simulink model "hpa_module"  (R2019a)
settings: Solver=FixedStepDiscrete  StartTime=0.0  StopTime=inf  RelTol=1e-3
InitFcn:
  | f = 300e6;
libraries: hdlsllib x5, simulink x1
settings Model: DataTypeOverride=Off  Creator=David Northcote  LastModifiedBy=David Northcote
settings DataIOCC: SaveOutput=off  SaveTime=off
settings OptimizationCC: BlockReduction=off  ConditionallyExecuteInputs=off  DefaultParameterBehavior=Inlined
settings DebuggingCC: AlgebraicLoopMsg=error  SingleTaskRateTransMsg=error
settings HardwareCC: ProdBitPerPointer=32  ProdBitPerSizeT=32  ProdBitPerPtrDiffT=32  ProdLargestAtomicFloat=None  ProdIntDivRoundTo=Undefined  ProdEndianess=Unspecified  ProdWordSize=32  ProdHWDeviceType=ASIC/FPGA->ASIC/FPGA  TargetBitPerPointer=64  TargetBitPerSizeT=64  TargetBitPerPtrDiffT=64  TargetLongLongMode=on  TargetIntDivRoundTo=Zero  TargetEndianess=LittleEndian  TargetWordSize=64  TargetHWDeviceType=Custom Processor->MATLAB Host Computer  ProdEqTarget=off

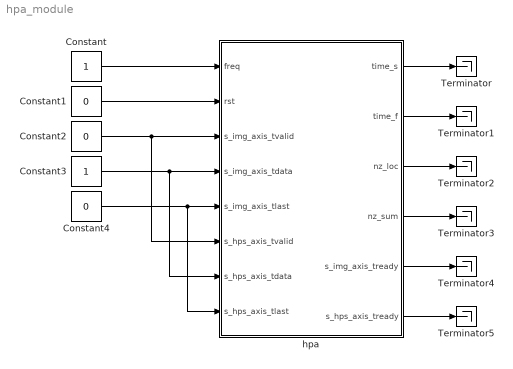
== system hpa_module ==
  Constant : Constant  OutDataTypeStr=uint32  SampleTime=1/f
  Constant1 : Constant  Value=0  OutDataTypeStr=boolean  SampleTime=1/f
  Constant2 : Constant  Value=0  OutDataTypeStr=boolean  SampleTime=1/f
  Constant3 : Constant  OutDataTypeStr=uint32  SampleTime=1/f
  Constant4 : Constant  Value=0  OutDataTypeStr=boolean  SampleTime=1/f
  Terminator{,1..5} (6 alike) : Terminator
  hpa : Subsystem  TreatAsAtomicUnit=on
  wires:
  Constant/1 -> hpa/1(freq)
  Constant1/1 -> hpa/2(rst)
  Constant2/1 -> hpa/6(s_hps_axis_tvalid), hpa/3(s_img_axis_tvalid)
  Constant3/1 -> hpa/7(s_hps_axis_tdata), hpa/4(s_img_axis_tdata)
  Constant4/1 -> hpa/8(s_hps_axis_tlast), hpa/5(s_img_axis_tlast)
  hpa/1(time_s) -> Terminator/1
  hpa/2(time_f) -> Terminator1/1
  hpa/3(nz_loc) -> Terminator2/1
  hpa/4(nz_sum) -> Terminator3/1
  hpa/6(s_hps_axis_tready) -> Terminator5/1
  hpa/5(s_img_axis_tready) -> Terminator4/1

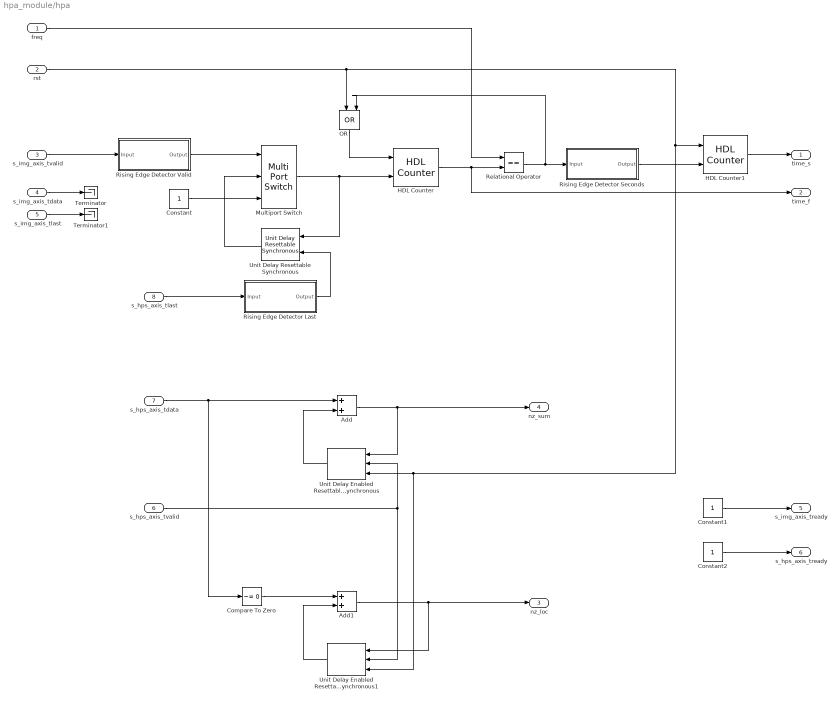
== system hpa_module/hpa ==
  freq : Inport
  rst : Inport  Port=2
  s_img_axis_tvalid : Inport  Port=3
  s_img_axis_tdata : Inport  Port=4
  s_img_axis_tlast : Inport  Port=5
  s_hps_axis_tvalid : Inport  Port=6
  s_hps_axis_tdata : Inport  Port=7
  s_hps_axis_tlast : Inport  Port=8
  Add : Sum  OutDataTypeStr=uint32
  Add1 : Sum  OutDataTypeStr=uint32
  Compare To Zero : simulink/Logic and Bit Operations/Compare To Zero  relop=~=  OutDataTypeStr=boolean
  Constant : Constant  OutDataTypeStr=boolean  SampleTime=-1
  Constant1 : Constant  OutDataTypeStr=boolean  SampleTime=1/f
  Constant2 : Constant  OutDataTypeStr=boolean  SampleTime=1/f
  HDL Counter : hdlsllib/Sources/HDL Counter  CountType=Free running  CountInit=0  CountStep=1  CountMax=25  CountFromType=Initial value  CountFrom=0  CountResetPort=on  CountLoadPort=off  CountEnbPort=on  CountDirPort=off  CountDataType=Unsigned  CountWordLen=32  CountFracLen=0  CountSampTime=1
      settings: SourceProductName=Simulink
  HDL Counter1 : hdlsllib/Sources/HDL Counter  CountType=Free running  CountInit=0  CountStep=1  CountMax=25  CountFromType=Initial value  CountFrom=0  CountResetPort=on  CountLoadPort=off  CountEnbPort=on  CountDirPort=off  CountDataType=Unsigned  CountWordLen=32  CountFracLen=0  CountSampTime=1
      settings: SourceProductName=Simulink
  Multiport Switch : MultiPortSwitch  DataPortOrder=Zero-based contiguous  Inputs=2  zeroidx=on
  OR : Logic  Operator=OR  IconShape=distinctive  AllPortsSameDT=off  OutDataTypeStr=boolean
  Relational Operator : RelationalOperator  Operator===  OutDataTypeStr=boolean  RndMeth=Simplest
  Rising Edge Detector Last : Subsystem
  Rising Edge Detector Seconds : Subsystem
  Rising Edge Detector Valid : Subsystem
  Terminator : Terminator
  Terminator1 : Terminator
  Unit Delay Enabled Resettable Synchronous : hdlsllib/Discrete/Unit Delay Enabled Resettable Synchronous  InitialCondition=0.0  SampleTime=-1
      settings: SourceProductName=Simulink  SourceProductBaseCode=SL
  Unit Delay Enabled Resettable Synchronous1 : hdlsllib/Discrete/Unit Delay Enabled Resettable Synchronous  InitialCondition=0.0  SampleTime=-1
      settings: SourceProductName=Simulink  SourceProductBaseCode=SL
  Unit Delay Resettable Synchronous : hdlsllib/Discrete/Unit Delay Resettable Synchronous  InitialCondition=0.0  SampleTime=-1
      settings: SourceProductName=Simulink  SourceProductBaseCode=SL
  time_s : Outport
  time_f : Outport  Port=2
  nz_loc : Outport  Port=3
  nz_sum : Outport  Port=4
  s_img_axis_tready : Outport  Port=5
  s_hps_axis_tready : Outport  Port=6
  wires:
  Multiport Switch/1 -> HDL Counter/2, Unit Delay Resettable Synchronous/1
  s_hps_axis_tlast/1 -> Rising Edge Detector Last/1(Input)
  Unit Delay Resettable Synchronous/1 -> Multiport Switch/2
  Constant/1 -> Multiport Switch/3
  s_img_axis_tvalid/1 -> Rising Edge Detector Valid/1(Input)
  Rising Edge Detector Valid/1(Output) -> Multiport Switch/1
  Relational Operator/1 -> OR/2, Rising Edge Detector Seconds/1(Input)
  HDL Counter/1 -> time_f/1, Relational Operator/2
  freq/1 -> Relational Operator/1
  HDL Counter1/1 -> time_s/1
  s_img_axis_tdata/1 -> Terminator/1
  s_img_axis_tlast/1 -> Terminator1/1
  Rising Edge Detector Seconds/1(Output) -> HDL Counter1/2
  OR/1 -> HDL Counter/1
  s_hps_axis_tdata/1 -> Compare To Zero/1, Add/1
  Add/1 -> nz_sum/1, Unit Delay Enabled Resettable Synchronous/1
  Unit Delay Enabled Resettable Synchronous/1 -> Add/2
  s_hps_axis_tvalid/1 -> Unit Delay Enabled Resettable Synchronous/2, Unit Delay Enabled Resettable Synchronous1/2
  Unit Delay Enabled Resettable Synchronous1/1 -> Add1/2
  Add1/1 -> nz_loc/1, Unit Delay Enabled Resettable Synchronous1/1
  Compare To Zero/1 -> Add1/1
  rst/1 -> OR/1, Unit Delay Enabled Resettable Synchronous1/3, Unit Delay Enabled Resettable Synchronous/3, HDL Counter1/1
  Rising Edge Detector Last/1(Output) -> Unit Delay Resettable Synchronous/2
  Constant1/1 -> s_img_axis_tready/1
  Constant2/1 -> s_hps_axis_tready/1

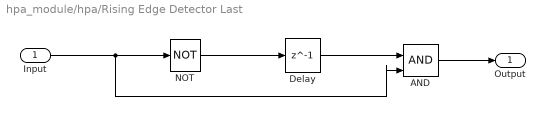
== system hpa_module/hpa/Rising Edge Detector Last ==
  Input : Inport
  AND : Logic  IconShape=distinctive  AllPortsSameDT=off  OutDataTypeStr=boolean
  Delay : Delay  DelayLength=1
  NOT : Logic  Operator=NOT  IconShape=distinctive  AllPortsSameDT=off  OutDataTypeStr=boolean
  Output : Outport
  wires:
  Input/1 -> NOT/1, AND/2
  AND/1 -> Output/1
  Delay/1 -> AND/1
  NOT/1 -> Delay/1

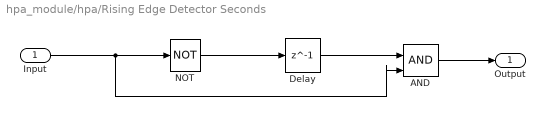
== system hpa_module/hpa/Rising Edge Detector Seconds ==
  Input : Inport
  AND : Logic  IconShape=distinctive  AllPortsSameDT=off  OutDataTypeStr=boolean
  Delay : Delay  DelayLength=1
  NOT : Logic  Operator=NOT  IconShape=distinctive  AllPortsSameDT=off  OutDataTypeStr=boolean
  Output : Outport
  wires:
  Input/1 -> NOT/1, AND/2
  AND/1 -> Output/1
  Delay/1 -> AND/1
  NOT/1 -> Delay/1

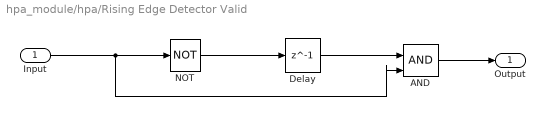
== system hpa_module/hpa/Rising Edge Detector Valid ==
  Input : Inport
  AND : Logic  IconShape=distinctive  AllPortsSameDT=off  OutDataTypeStr=boolean
  Delay : Delay  DelayLength=1
  NOT : Logic  Operator=NOT  IconShape=distinctive  AllPortsSameDT=off  OutDataTypeStr=boolean
  Output : Outport
  wires:
  NOT/1 -> Delay/1
  Delay/1 -> AND/1
  AND/1 -> Output/1
  Input/1 -> AND/2, NOT/1
